simulink model "path_estimation_2"  (R2023b)
settings: Solver=VariableStepAuto  StartTime=0.0  StopTime=10.0  RelTol=1e-3
libraries: dspadpt3 x3, dspsrcs4 x1
settings Model: Creator=mykni  LastModifiedBy=mykni

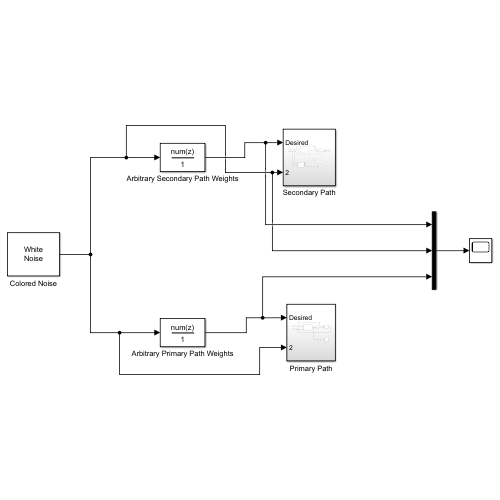
[thumbnail: Simulink's stored preview of the top-level diagram]
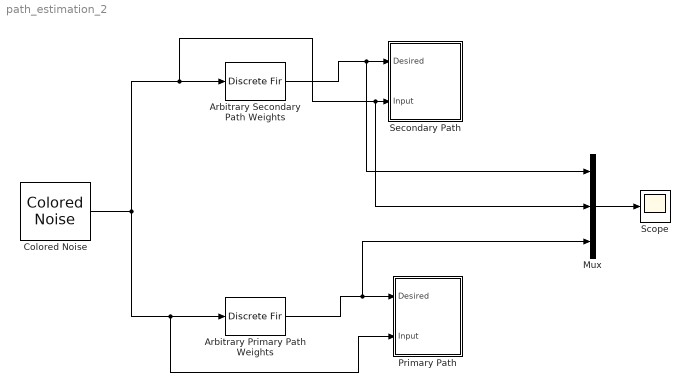
== system path_estimation_2 ==
  Arbitrary Primary Path Weights : DiscreteFir  Coefficients=conv([.1 -.1 .2 -.2 .3 -.3 .15 -.15],[0.5 0.5 -.3 -.3 -.2 -.2])
  Arbitrary Secondary Path Weights : DiscreteFir  Coefficients=[0.5 0.5 -.3 -.3 -.2 -.2]
  Colored Noise : dspsrcs4/Colored Noise  Color=white  InverseFrequencyPower=1  BoundedOutput=on  NumChannels=1  OutputDataType=double  SamplesPerFrame=1  SampleTime=1/41000  RandomStream=mt19937ar with seed  Seed=67  SimulateUsing=Interpreted execution
      settings: LibrarySourceBlock=audiosources/Colored Noise
  Mux : Mux  Inputs=3
  Primary Path : Subsystem
  Scope : Scope
  Secondary Path : Subsystem
  wires:
  Colored Noise/1 -> Primary Path/2(Input), Arbitrary Primary Path Weights/1, Mux/2, Secondary Path/2(Input), Arbitrary Secondary Path Weights/1
  Arbitrary Secondary Path Weights/1 -> Mux/1, Secondary Path/1(Desired)
  Arbitrary Primary Path Weights/1 -> Mux/3, Primary Path/1(Desired)
  Mux/1 -> Scope/1

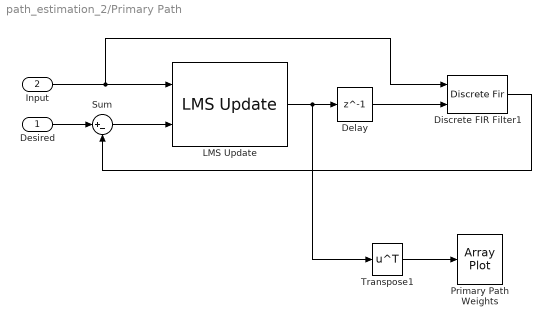
== system path_estimation_2/Primary Path ==
  Desired : Inport
  Input : Inport  Port=2
  Delay : Delay  DelayLength=1  InitialCondition=0
  Discrete FIR Filter1 : DiscreteFir  CoefSource=Input port
      settings: InputPortMap=u0,u1
  LMS Update : dspadpt3/LMS Update  Method=Normalized LMS  Length=32  NumFilters=1  StepSizeSource=Property  StepSize=0.2  LeakageFactor=1.0  InitialConditions=0  AdaptiveFilterMode=Tapped delay-line FIR filter  EnableAdaptInput=off  EnableResetInput=off  SimulateUsing=Code generation
  Primary Path Weights : ArrayPlot  WindowPosition=[2.000000,50.000000,766.000000,785.000000,]  ScopeFrameLocation=window  YLimits=[-0.0074 0.0219]
  Sum : Sum  Inputs=|+-
  Transpose1 : Math  Operator=transpose
  wires:
  Discrete FIR Filter1/1 -> Sum/2
  Delay/1 -> Discrete FIR Filter1/2
  Transpose1/1 -> Primary Path Weights/1
  LMS Update/1 -> Transpose1/1, Delay/1
  Input/1 -> Discrete FIR Filter1/1, LMS Update/1
  Sum/1 -> LMS Update/2
  Desired/1 -> Sum/1

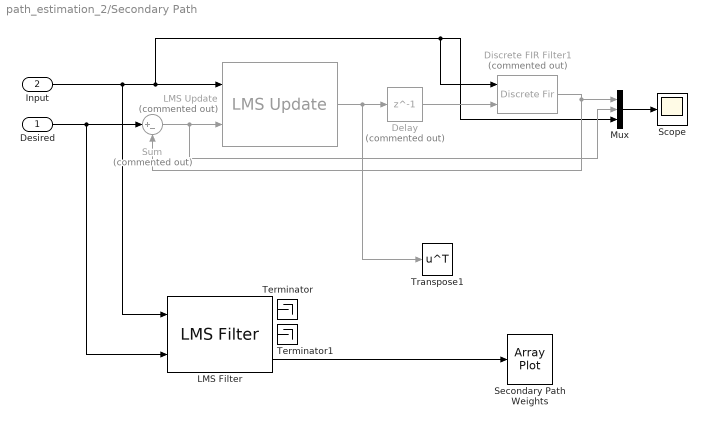
== system path_estimation_2/Secondary Path ==
  Desired : Inport
  Input : Inport  Port=2
  Delay : Delay  Commented=on  DelayLength=1  InitialCondition=0
  Discrete FIR Filter1 : DiscreteFir  Commented=on  CoefSource=Input port
      settings: InputPortMap=u0,u1
  LMS Filter : dspadpt3/LMS Filter  Algo=Normalized LMS  L=32  stepflag=Dialog  mu=0.2  leakage=1.0  ic=0  Adapt=off  resetflag=None  weights=on  addnparflag=off  roundingMode=Floor  overflowMode=off  secondCoeffMode=Binary point scaling  secondCoeffWordLength=2  secondCoeffFracLength=15  prodOutput2Mode=Binary point scaling  prodOutput2FracLength=20  prodOutput3Mode=Binary point scaling  prodOutput3FracLength=20  prodOutput4Mode=Binary point scaling  prodOutput4FracLength=20  quotientMode=Binary point scaling  quotientFracLength=20  accum2Mode=Binary point scaling  accum2FracLength=20
      settings: LibrarySourceBlock=dsphdlsupportfiltering/LMS Filter
  LMS Update : dspadpt3/LMS Update  Commented=on  Method=Normalized LMS  Length=32  NumFilters=1  StepSizeSource=Property  StepSize=0.2  LeakageFactor=1.0  InitialConditions=0  AdaptiveFilterMode=Tapped delay-line FIR filter  EnableAdaptInput=off  EnableResetInput=off  SimulateUsing=Code generation
  Mux : Mux  Inputs=3
  Scope : Scope
  Secondary Path Weights : ArrayPlot  WindowPosition=[770.000000,50.000000,766.000000,785.000000,]  ScopeFrameLocation=window  YLimits=[-0.0714 0.2783]
  Sum : Sum  Commented=on  Inputs=|+-
  Terminator : Terminator
  Terminator1 : Terminator
  Transpose1 : Math  Operator=transpose
  wires:
  Desired/1 -> LMS Filter/2, Sum/1
  Input/1 -> LMS Filter/1, Mux/3, Discrete FIR Filter1/1, LMS Update/1
  Delay/1 -> Discrete FIR Filter1/2
  LMS Update/1 -> Transpose1/1, Delay/1
  Sum/1 -> Mux/2, LMS Update/2
  Discrete FIR Filter1/1 -> Mux/1, Sum/2
  Mux/1 -> Scope/1
  LMS Filter/3 -> Secondary Path Weights/1
